simulink subsystem "closedLoopFuzzyPI"  (R2021a)
settings: Solver=VariableStepAuto  StartTime=0.0  StopTime=10.0  RelTol=1e-3
libraries: fuzblock x1
settings Model: Creator=vash  LastModifiedBy=vash

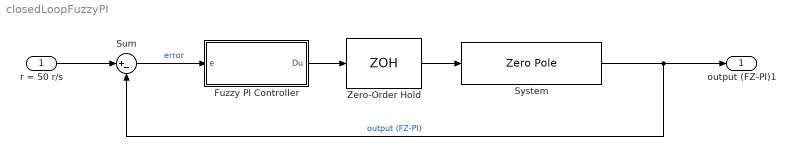
== system closedLoopFuzzyPI ==
  r = 50 r/s : Inport
  Fuzzy PI Controller : Subsystem  TreatAsAtomicUnit=on
  Sum : Sum  Inputs=|+-
  System : ZeroPole  Zeros=[]  Poles=[-0.1 -10]  Gain=25
  Zero-Order Hold : ZeroOrderHold  SampleTime=-1
  output (FZ-PI)1 : Outport
  wires:
  Sum/1 -> Fuzzy PI Controller/1(e)  "error"
  System/1 -> output (FZ-PI)1/1, Sum/2  "output (FZ-PI)"
  Fuzzy PI Controller/1(Du) -> Zero-Order Hold/1
  Zero-Order Hold/1 -> System/1
  r = 50 r/s/1 -> Sum/1

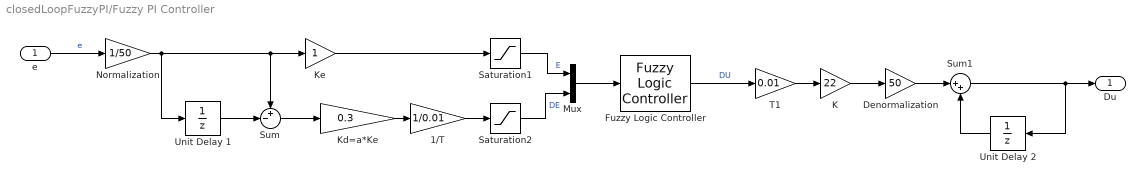
== system closedLoopFuzzyPI/Fuzzy PI Controller ==
  e : Inport
  1/T : Gain  Gain=1/0.01
  Denormalization : Gain  Gain=50
  Fuzzy Logic Controller : fuzblock/Fuzzy Logic  Controller  FIS='flc.fis'  OutputSampleNumber=101  DataType=double  FuzzifiedInputs=off  RuleFiringStrengths=off  RuleOutputs=off  AggregatedOutputs=off  SimulateUsing=Interpreted execution  OutOfRangeInputValueMessage=warning  NoRuleFiredMessage=warning  EmptyOutputFuzzySetMessage=warning
  K : Gain  Gain=22
  Kd=a*Ke : Gain  Gain=0.3
  Ke : Gain
  Mux : Mux  Inputs=2
  Normalization : Gain  Gain=1/50
  Saturation1 : Saturate  UpperLimit=1  LowerLimit=-1  ZeroCross=off  OutMin=[-1]  OutMax=[1]  RndMeth=Round
  Saturation2 : Saturate  UpperLimit=1  LowerLimit=-1  ZeroCross=off  OutMin=[-1]  OutMax=[1]  RndMeth=Round
  Sum : Sum  Inputs=+-|
  Sum1 : Sum  Inputs=|++
  T1 : Gain  Gain=0.01
  Unit Delay 1 : UnitDelay  SampleTime=-1  HasFrameUpgradeWarning=on
  Unit Delay 2 : UnitDelay  SampleTime=-1  HasFrameUpgradeWarning=on
  Du : Outport
  wires:
  Mux/1 -> Fuzzy Logic Controller/1
  Unit Delay 2/1 -> Sum1/2
  Sum1/1 -> Du/1, Unit Delay 2/1
  Denormalization/1 -> Sum1/1
  K/1 -> Denormalization/1
  T1/1 -> K/1
  Saturation2/1 -> Mux/2  "DE"
  Saturation1/1 -> Mux/1  "E"
  1/T/1 -> Saturation2/1
  Kd=a*Ke/1 -> 1/T/1
  Sum/1 -> Kd=a*Ke/1
  Ke/1 -> Saturation1/1
  Unit Delay 1/1 -> Sum/2
  Normalization/1 -> Ke/1, Sum/1, Unit Delay 1/1
  Fuzzy Logic Controller/1 -> T1/1  "DU"
  e/1 -> Normalization/1  "e"
